simulink model "WareHouseTaskRobotSimulationModel_FaultModel"  (R2024b)
settings: Solver=FixedStepAuto  StartTime=0.0  StopTime=30  RelTol=1e-3  EnableMultiTasking=on
settings Model: Creator=marcob  LastModifiedBy=marcob
settings DebuggingCC: InheritedTsInSrcMsg=none

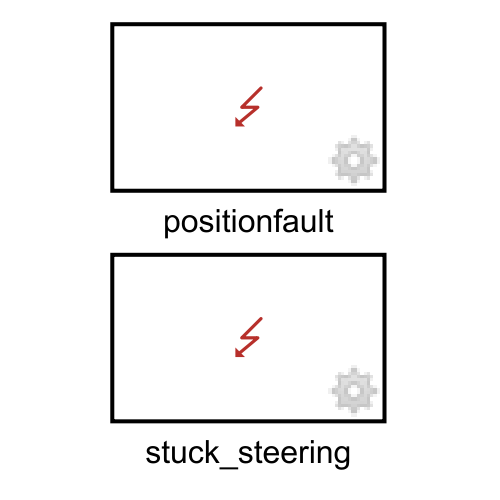
[thumbnail: Simulink's stored preview of the top-level diagram]
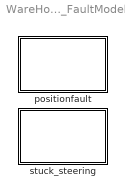
== system WareHouseTaskRobotSimulationModel_FaultModel ==
  positionfault : Subsystem  TreatAsAtomicUnit=on  IsInjectorSS=on
  stuck_steering : Subsystem  TreatAsAtomicUnit=on  IsInjectorSS=on

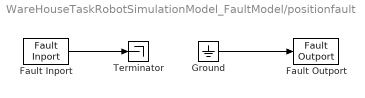
== system WareHouseTaskRobotSimulationModel_FaultModel/positionfault ==
  Fault Inport : FaultInport
  Fault Outport : FaultOutport
  Ground : Ground
  Terminator : Terminator
  wires:
  Ground/1 -> Fault Outport/1
  Fault Inport/1 -> Terminator/1

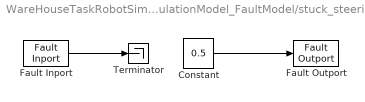
== system WareHouseTaskRobotSimulationModel_FaultModel/stuck_steering ==
  Constant : Constant  Value=0.5
  Fault Inport : FaultInport
  Fault Outport : FaultOutport
  Terminator : Terminator
  wires:
  Constant/1 -> Fault Outport/1
  Fault Inport/1 -> Terminator/1
